simulink model "accelerometer"  (R2018a)
settings: Solver=FixedStepAuto  StartTime=0.0  StopTime=10.0  FixedStep=0.0001  RelTol=1e-3
libraries: simulink_extras x3
settings Model: Creator=David  LastModifiedBy=David

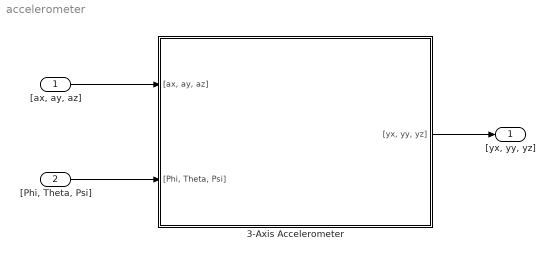
== system accelerometer ==
  "[ax, ay, az]" : Inport
  "[Phi, Theta, Psi]" : Inport  Port=2
  3-Axis Accelerometer : Subsystem  mask{g=9.81, SampleTime=0.01, accelXNoiseDensity=0.1/sqrt(100), accelYNoiseDensity=0.1/sqrt(100), accelZNoiseDensity=0.1/sqrt(100), accelXBandwidthHz=1000, accelYBandwidthHz=1000, accelZBandwidthHz=1000, accelXInit=0, accelYInit=0, accelZInit=0, accelXUpperSaturation=inf, accelXLowerSaturation=-inf, accelYUpperSaturation=inf, accelYLowerSaturation=-inf, accelZUpperSaturation=inf, accelZLowerSaturation=-inf, accelXResolution=1E-12, accelYResolution=1E-12, accelZResolution=1E-12}
      mask prompts: g "Gravity (m/s^2)"; SampleTime "Accelerometer Sample Time (s)"; accelXNoiseDensity "X Accelerometer Noise Density (m/s^2/sqrt(Hz))"; accelYNoiseDensity "Y Accelerometer Noise Density (m/s^2/sqrt(Hz))"; accelZNoiseDensity "Z Accelerometer Noise Density (m/s^2/sqrt(Hz))"; accelXBandwidthHz "X Accelerometer Bandwidth (Hz)"; accelYBandwidthHz "Y Accelerometer Bandwidth (Hz)"; accelZBandwidthHz "Z Accelerometer Bandwidth (Hz)"; accelXInit "X Accelerometer Initial Condition (m/s^2)"; accelYInit "Y Accelerometer Initial Condition (m/s^2)"; accelZInit "Z Accelerometer Initial Condition (m/s^2)"; accelXUpperSaturation "X Accelerometer Measurement Upper Saturation Limit (m/s^2)"; accelXLowerSaturation "X Accelerometer Measurement Lower Saturation Limit (m/s^2)"; accelYUpperSaturation "Y Accelerometer Measurement Upper Saturation Limit (m/s^2)"; accelYLowerSaturation "Y Accelerometer Measurement Lower Saturation Limit (m/s^2)"; accelZUpperSaturation "Z Accelerometer Measurement Upper Saturation Limit (m/s^2)"; accelZLowerSaturation "Z Accelerometer Measurement Upper Saturation Limit (m/s^2)"; accelXResolution "X Accelerometer Resolution (m/s^2)"; accelYResolution "Y Accelerometer Resolution (m/s^2)"; accelZResolution "Z Accelerometer Resolution (m/s^2)"
      mask DialogControl DescGroupVar Prompt: MEMS Accelerometer Model
      mask DialogControl DescTextVar Prompt: MEMS Accelerometer Model with White Noise Modelling
      mask DialogControl Container7 Prompt: System Characteristics
      mask DialogControl Container4 Prompt: Noise Characteristics
      mask DialogControl Container8 Prompt: Density
      mask DialogControl Container10 Prompt: Sensor Dynamics
      mask DialogControl Container13 Prompt: Bandwidth
      mask DialogControl Container12 Prompt: Initial Conditions
      mask DialogControl Container15 Prompt: Limits and Quantization
      mask DialogControl Container17 Prompt: Limits
      mask DialogControl Container20 Prompt: Quantization
      mask DialogControl Control2 Prompt: This can be calculated with the following equation:
      mask DialogControl Control3 Prompt: Physical Resolution = measurement_span/(2^resolution_bits - 1)
      mask Display:
      | image('mems_accel.png')
      | 
      | color('red')
      | 
      | port_label('input', 1, '[a_x, a_y, a_z] (m/s^2)', 'texMode', 'on')
      | port_label('input', 2, '[\phi, \theta, \psi] (rad)', 'texMode', 'on')
      | 
      | port_label('output', 1, '[y_{accel_x}, y_{accel_y}, y_{accel_z}] (m/s^2)', 'texMode', 'on')
  "[yx, yy, yz]" : Outport
  wires:
  "[ax, ay, az]"/1 -> 3-Axis Accelerometer/1("[ax, ay, az]")
  "[Phi, Theta, Psi]"/1 -> 3-Axis Accelerometer/2("[Phi, Theta, Psi]")
  3-Axis Accelerometer/1("[yx, yy, yz]") -> "[yx, yy, yz]"/1

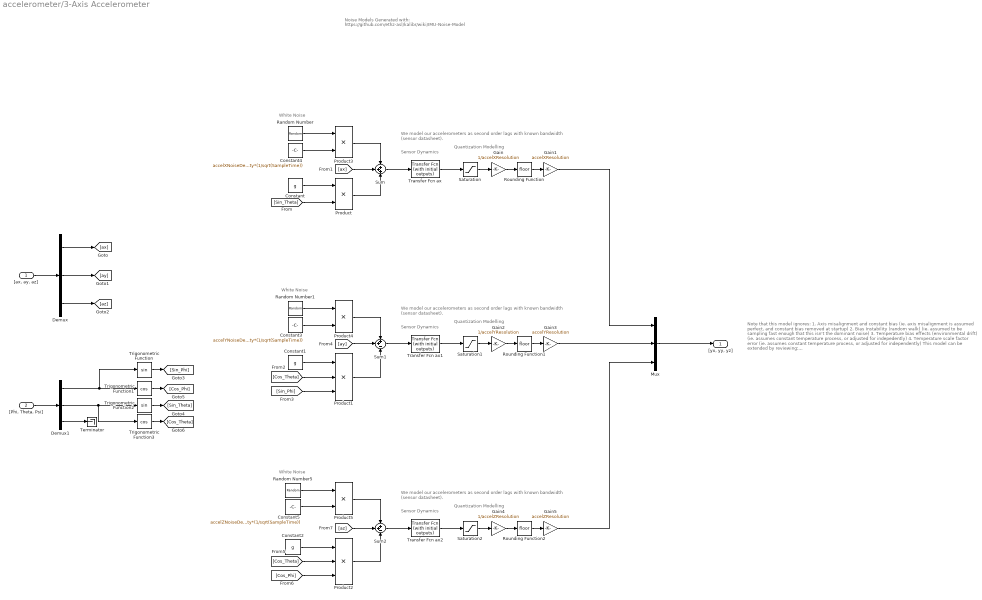
== system accelerometer/3-Axis Accelerometer ==
  note: Quantization Modelling
  note: Sensor Dynamics
  note: Note that this model ignores:
      | 1. Axis misalignment and constant bias (ie. axis misalignment is assumed perfect, and constant bias removed at startup)
      | 2. Bias Instability (random walk) (ie. assumed to be sampling fast enough that this isn't the dominant noise)
      | 3. Temperature bias effects (environmental drift) (ie. assumes constant temperature process, or adjusted for indepedently)
      | 4. Temperature scale factor error (ie. assumes constant temperature process, or adjusted for independently)
      |
      | This model can be extended by reviewing:
      | https://www.mathworks.com/help/fusion/ref/imusensor-system-object.html?searchHighlight=imuSensor&s_tid=doc_srchtitle
  note: We model our accelerometers as second order lags with known bandwidth
      | (sensor datasheet).
  note: White Noise
  note: Noise Models Generated with:
      | https://github.com/ethz-asl/kalibr/wiki/IMU-Noise-Model
  note: White Noise
  note: White Noise
  note: We model our accelerometers as second order lags with known bandwidth
      | (sensor datasheet).
  note: Quantization Modelling
  note: Sensor Dynamics
  note: We model our accelerometers as second order lags with known bandwidth
      | (sensor datasheet).
  note: Quantization Modelling
  note: Sensor Dynamics
  "[ax, ay, az]" : Inport
  "[Phi, Theta, Psi]" : Inport  Port=2
  Constant : Constant  Value=g
  Constant1 : Constant  Value=g
  Constant2 : Constant  Value=g
  Constant3 : Constant  Value=accelYNoiseDensity*(1/sqrt(SampleTime))
  Constant4 : Constant  Value=accelXNoiseDensity*(1/sqrt(SampleTime))
  Constant5 : Constant  Value=accelZNoiseDensity*(1/sqrt(SampleTime))
  Demux : Demux  Outputs=3
  Demux1 : Demux  Outputs=3
  Gain : Gain  Gain=1/accelXResolution
  Gain1 : Gain  Gain=accelXResolution
  Gain2 : Gain  Gain=1/accelYResolution
  Gain3 : Gain  Gain=accelYResolution
  Gain4 : Gain  Gain=1/accelZResolution
  Gain5 : Gain  Gain=accelZResolution
  Mux : Mux  Inputs=3
  Product{,3..5} (4 alike) : Product
  Product1 : Product  Inputs=3
  Product2 : Product  Inputs=3
  Random Number : RandomNumber  SampleTime=SampleTime
  Random Number1 : RandomNumber  SampleTime=SampleTime
  Random Number5 : RandomNumber  SampleTime=SampleTime
  Rounding Function : Rounding
  Rounding Function1 : Rounding
  Rounding Function2 : Rounding
  Saturation : Saturate  UpperLimit=accelXUpperSaturation  LowerLimit=accelXLowerSaturation  ZeroCross=off
  Saturation1 : Saturate  UpperLimit=accelYUpperSaturation  LowerLimit=accelYLowerSaturation  ZeroCross=off
  Saturation2 : Saturate  UpperLimit=accelZUpperSaturation  LowerLimit=accelZLowerSaturation  ZeroCross=off
  Sum : Sum  Inputs=+++
  Sum1 : Sum  Inputs=++-
  Sum2 : Sum  Inputs=++-
  Terminator : Terminator
  Transfer Fcn ax : simulink_extras/Additional Linear/Transfer Fcn (with initial outputs)  N=[(accelXBandwidthHz*2*pi)^2]  D="[1,  2*accelXBandwidthHz*2*pi, (accelXBandwidthHz*2*pi)^2]"  Y0=accelXInit  U0=accelXInit
  Transfer Fcn ax1 : simulink_extras/Additional Linear/Transfer Fcn (with initial outputs)  N=[(accelYBandwidthHz*2*pi)^2]  D="[1,  2*accelYBandwidthHz*2*pi, (accelYBandwidthHz*2*pi)^2]"  Y0=accelXInit  U0=accelXInit
  Transfer Fcn ax2 : simulink_extras/Additional Linear/Transfer Fcn (with initial outputs)  N=[(accelZBandwidthHz*2*pi)^2]  D="[1,  2*accelZBandwidthHz*2*pi, (accelZBandwidthHz*2*pi)^2]"  Y0=accelXInit  U0=accelXInit
  Trigonometric Function : Trigonometry
  Trigonometric Function1 : Trigonometry  Operator=cos
  Trigonometric Function2 : Trigonometry
  Trigonometric Function3 : Trigonometry  Operator=cos
  "[yx, yy, yz]" : Outport
  wires:
  Product/1 -> Sum/3
  [ax] -> Sum/2
  Trigonometric Function3/1 -> [Cos_Theta]
  Sum/1 -> Transfer Fcn ax/1
  Mux/1 -> "[yx, yy, yz]"/1
  [Cos_Phi] -> Product2/3
  Trigonometric Function2/1 -> [Sin_Theta]
  Constant2/1 -> Product2/1
  Demux1/1 -> Trigonometric Function1/1, Trigonometric Function/1
  Demux1/2 -> Trigonometric Function3/1, Trigonometric Function2/1
  [Sin_Theta] -> Product/2
  "[Phi, Theta, Psi]"/1 -> Demux1/1
  [Cos_Theta] -> Product2/2
  [az] -> Sum2/2
  [Cos_Theta] -> Product1/2
  Product2/1 -> Sum2/3
  Trigonometric Function/1 -> [Sin_Phi]
  [ay] -> Sum1/2
  Product1/1 -> Sum1/3
  [Sin_Phi] -> Product1/3
  Trigonometric Function1/1 -> [Cos_Phi]
  Constant1/1 -> Product1/1
  Constant/1 -> Product/1
  Demux1/3 -> Terminator/1
  "[ax, ay, az]"/1 -> Demux/1
  Random Number/1 -> Product3/1
  Constant4/1 -> Product3/2
  Constant3/1 -> Product4/2
  Constant5/1 -> Product5/2
  Demux/1 -> [ax]
  Demux/2 -> [ay]
  Demux/3 -> [az]
  Product3/1 -> Sum/1
  Product4/1 -> Sum1/1
  Random Number1/1 -> Product4/1
  Random Number5/1 -> Product5/1
  Product5/1 -> Sum2/1
  Saturation/1 -> Gain/1
  Transfer Fcn ax/1 -> Saturation/1
  Gain/1 -> Rounding Function/1
  Rounding Function/1 -> Gain1/1
  Gain1/1 -> Mux/1
  Gain2/1 -> Rounding Function1/1
  Saturation1/1 -> Gain2/1
  Transfer Fcn ax1/1 -> Saturation1/1
  Rounding Function1/1 -> Gain3/1
  Sum1/1 -> Transfer Fcn ax1/1
  Gain3/1 -> Mux/2
  Gain5/1 -> Mux/3
  Sum2/1 -> Transfer Fcn ax2/1
  Rounding Function2/1 -> Gain5/1
  Saturation2/1 -> Gain4/1
  Transfer Fcn ax2/1 -> Saturation2/1
  Gain4/1 -> Rounding Function2/1
